simulink model "TX_RX_ppm_test"  (R2018a)
settings: Solver=VariableStepAuto  StartTime=0.0  StopTime=5  RelTol=1e-3
undefined symbols (not defined in the file): startfcn_spectrum_analyzer
libraries: dspmlti4 x1, dspstat3 x1, sdrrlib x1, rtlsdr_book_library x1
settings Model: Creator=sun  LastModifiedBy=root

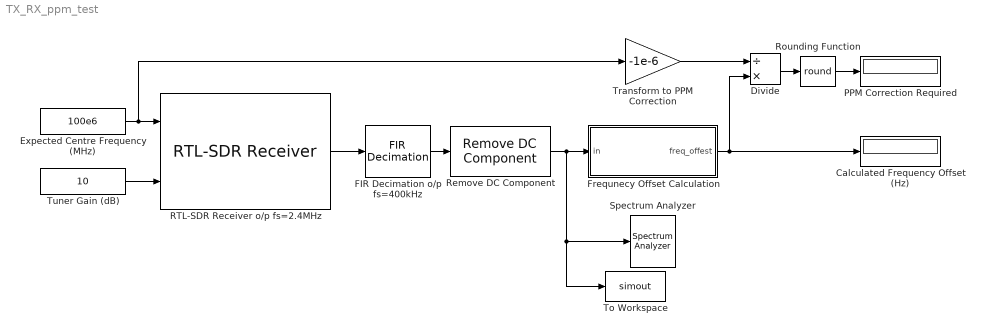
== system TX_RX_ppm_test ==
  " Calculated Frequency Offset (Hz)" : Display
      settings: Format=bank
  Divide : Product  Inputs=/*
  Expected Centre Frequency (MHz) : Constant  Value=100e6
  FIR Decimation o/p fs=400kHz : dspmlti4/FIR Decimation  FilterSource=Dialog parameters  h=fir1(100,0.3)  D=6  filtStruct=Direct form  FilterObject=Hm_firdecim  InputProcessing=Columns as channels (frame based)  framing=Allow multirate processing  inputOffset=0  outputBufInitCond=0  roundingMode=Floor  overflowMode=off  firstCoeffDataTypeStr=Inherit: Same word length as input  firstCoeffMin=[]  firstCoeffMax=[]  firstCoeffLastDataTypeStr=Inherit: Same word length as input  outputDataTypeStr=Inherit: Same as accumulator  outputMin=[]  outputMax=[]  outputLastDataTypeStr=Inherit: Same as accumulator
  Frequnecy Offset Calculation : Subsystem
  PPM Correction Required : Display
  RTL-SDR Receiver o/p fs=2.4MHz : sdrrlib/RTL-SDR Receiver  IPAddress=0  CenterFrequencySource=Input port  CenterFrequency=240e6  GainSource=Input port  Gain=0  ADCRate=2.4e6  FrequencyCorrection=13  LostSamplesOutputPort=off  LatencyOutputPort=off  OutputDataType=single  FrameLength=4096  EnableBurstMode=off  NumFramesInBurst=20  sobjType=sdrr.internal.SDRRTLReceiverSL  dataUDPPort=-1  ctrlUDPPort=-1  subDeviceList=nosubdev  sdrBlockType=SDRBlockTypeSLT.SDRRxBlock  requester=UNUSED_BY_SFCN  sdrExecutionMode=SDRExecutionModeSLT.ExecModeHW  BypassUserLogic=off  DecimatorSelect=DDC decimator  SourceSelect=RF data  SineAmplitude=16000  EnableInternalClock=off  BypassIQBalance=off  IFBandwidth=40e6  ADCRateSource=Dialog  IntermediateFrequency=0  DecimationFactorSource=Dialog  DecimationFactor=512  RFFrequencyIsTunable=logical(1)  SampleTime=(4096)/(2.4e6)  IFBandwidthSource=Dialog  SineFrequency=30000  BypassDCBlockingFilter=off  IntermediateFrequencySource=Dialog  IQBalanceCoefficients=64  SkipAllHardwareResetAndInitialization=off  EnableIQCalibrationTable=on  CacheIQCalibrationTable=off  EnableOffsetTuning=off  EnableRTLAGC=off  EnableTestMode=off  EnableTunerAGC=off  FrequencyCorrectionSource=Dialog  NumMLBuffers=128  NumUSBBuffers=16  RTLCrystalFrequency=28800000  TunerCrystalFrequency=28800000
      settings: SourceProductName=Communications System Toolbox Support Package for RTL-SDR Radio  SourceProductBaseCode=RTLSDR
  Remove DC Component : rtlsdr_book_library/Additional Tools/Remove DC Component
      settings: SourceProductName=RTL-SDR Book Library
  Rounding Function : Rounding  Operator=round
  Spectrum Analyzer : SpectrumAnalyzer  StartFcn=startfcn_spectrum_analyzer;
  To Workspace : ToWorkspace  VariableName=simout  SaveFormat=Timeseries  SampleTime=-1
  Transform to PPM Correction : Gain  Gain=-1e-6
  Tuner Gain (dB) : Constant  Value=10
  wires:
  Divide/1 -> Rounding Function/1
  FIR Decimation o/p fs=400kHz/1 -> Remove DC Component/1
  Rounding Function/1 -> PPM Correction Required/1
  Transform to PPM Correction/1 -> Divide/1
  Remove DC Component/1 -> Frequnecy Offset Calculation/1(in), To Workspace/1, Spectrum Analyzer/1
  RTL-SDR Receiver o/p fs=2.4MHz/1 -> FIR Decimation o/p fs=400kHz/1
  Frequnecy Offset Calculation/1(freq_offest) -> " Calculated Frequency Offset (Hz)"/1, Divide/2
  Expected Centre Frequency (MHz)/1 -> RTL-SDR Receiver o/p fs=2.4MHz/1, Transform to PPM Correction/1
  Tuner Gain (dB)/1 -> RTL-SDR Receiver o/p fs=2.4MHz/2

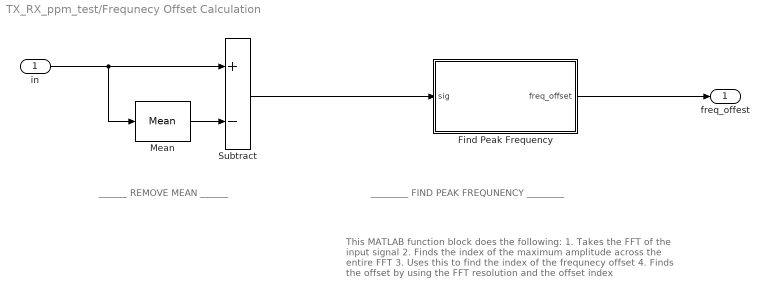
== system TX_RX_ppm_test/Frequnecy Offset Calculation ==
  note: This MATLAB function block does the following:
      | 1. Takes the FFT of the input signal
      | 2.  Finds the index of the maximum amplitude across the entire FFT
      | 3.  Uses this to find the index of the frequnecy offset
      | 4.  Finds the offset by using the FFT resolution and the offset index
  note: ______ REMOVE MEAN ______
  note: ________ FIND PEAK FREQUNENCY ________
  in : Inport
  Find Peak Frequency : MATLAB Function  TreatAsAtomicUnit=on
  Mean : dspstat3/Mean  run=off  InputProcessing=Columns as channels (frame based)  reset_popup=None  directionMode=Each column  dimension=1  roiEnable=off  roiType=Rectangles  roiPortion=Entire ROI  roiOutput=Individual statistics for each ROI  roiFlag=off  roundingMode=Floor  overflowMode=off  outputDataTypeStr=Inherit: Same as accumulator  outputMin=[]  outputMax=[]  outputLastDataTypeStr=Inherit: Same as accumulator
  Subtract : Sum  Inputs=+-
  freq_offest : Outport
  wires:
  Mean/1 -> Subtract/2
  in/1 -> Subtract/1, Mean/1
  Subtract/1 -> Find Peak Frequency/1(sig)
  Find Peak Frequency/1(freq_offset) -> freq_offest/1

== matlab function TX_RX_ppm_test/Frequnecy Offset Calculation/Find Peak Frequency ==
  data: freq_offset output; sig input
function freq_offset  = fcn(sig)

nfft = 8192;                        % length of FFT
fs = 400e3;                         % sampling frequency
delta_f = fs/nfft;                  % frequency resolution of FFT // width of fft bin

fft_sig = fft(sig,nfft);            % find fft of signal [ +ve freqs , -ve freqs ]
fft_sig = fftshift(fft_sig);        % rearrange to be [ -ve freqs , +ve freqs ]

[~, max_idx] = max(fft_sig);        % find index of max component in fft 
offset_idx = max_idx-1-nfft/2;      % convert to index symmetric with 0
freq_offset = offset_idx*delta_f;   % map offset index back to frequency

end
